simulink model "BPSK_modulation"  (Simulink 8.1)
settings: Solver=ode45  StartTime=0.0  StopTime=10.0  RelTol=1e-3
undefined symbols (not defined in the file or in its folder): get
libraries: commsink2 x1, commrandsrc2 x1
settings Model: Creator=User  LastModifiedBy=Viet
settings DataIOCC: SignalLoggingSaveFormat=Dataset
settings OptimizationCC: ExpressionDepthLimit=128
settings DebuggingCC: FcnCallInpInsideContextMsg=EnableAllAsError
settings GRTTargetCC: CombineOutputUpdateFcns=on  GRTInterface=off

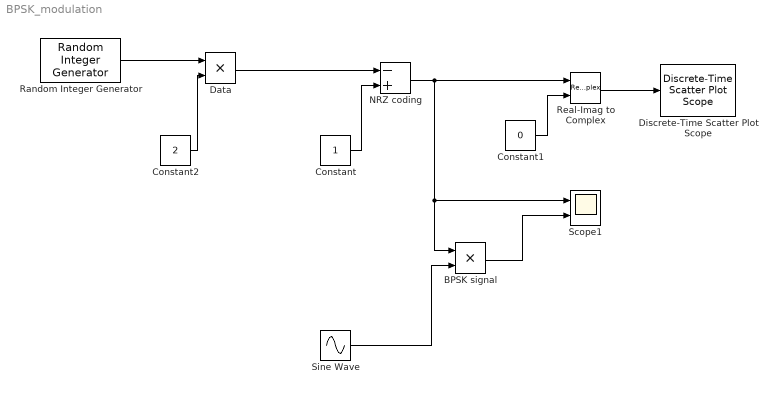
== system BPSK_modulation ==
  BPSK signal : Product
  Constant : Constant
  Constant1 : Constant  Value=0
  Constant2 : Constant  Value=2
  Data : Product
  Discrete-Time Scatter Plot Scope : commsink2/Discrete-Time Scatter Plot Scope  Tag=ScatterPlot  sampPerSymb=1  offsetEye=0  numTraces=40  numNewFrames=40  LineMarkers=*  LineColors=b  fading=on  render=on  AxisGrid=on  xMin=-3.3  xMax=3.315  yMin=-3.3  yMax=3.315  inphaseLabel=In-phase Amplitude  quadratureLabel=Quadrature Amplitude  openScopeAtSimStart=on  FrameNumber=off  FigPos=get(0,'defaultfigureposition');  figTitle=Scatter Plot  numLinesMax=8  block_type_=scatter
  NRZ coding : Sum  Inputs=-+
  Random Integer Generator : commrandsrc2/Random Integer Generator  mul=2  seed=37  Ts=1/10  frameBased=off  sampPerFrame=1  orient=off  outDataType=double
  Real-Imag to Complex : RealImagToComplex
  Scope1 : Scope  NumInputPorts=2
      settings: TickLabels=on  ShowLegends=on  TimeRange=2  YMin=-2~-2  YMax=2~2
  Sine Wave : Sin  Frequency=20*pi  SampleTime=0.001
  wires:
  Sine Wave/1 -> BPSK signal/2
  Real-Imag to Complex/1 -> Discrete-Time Scatter Plot Scope/1
  BPSK signal/1 -> Scope1/2
  Constant1/1 -> Real-Imag to Complex/2
  Random Integer Generator/1 -> Data/1
  Constant2/1 -> Data/2
  Data/1 -> NRZ coding/1
  Constant/1 -> NRZ coding/2
  NRZ coding/1 -> Scope1/1, BPSK signal/1, Real-Imag to Complex/1
